simulink model "mavlinkMST"  (R2025b)
settings: Solver=ode1  StartTime=0.0  StopTime=inf  FixedStep=0.01  RelTol=1e-3
libraries: instrumentlib x2, uavmavlinklib x1
settings Model: Creator=y3353li  LastModifiedBy=yangli
settings DebuggingCC: UnderspecifiedInitializationDetection=Classic  MergeDetectMultiDrivingBlocksExec=none
settings ModelReferenceCC: PropagateSignalLabelsOutOfModel=off

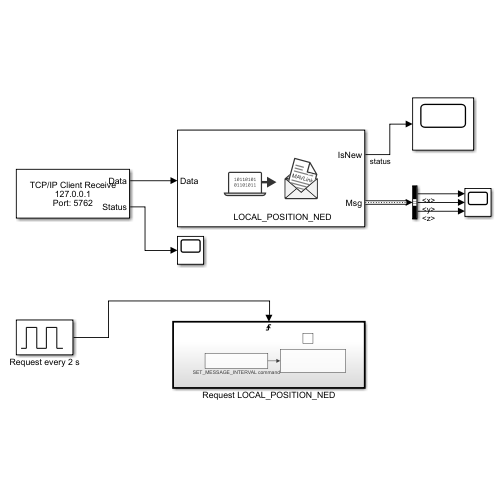
[thumbnail: Simulink's stored preview of the top-level diagram]
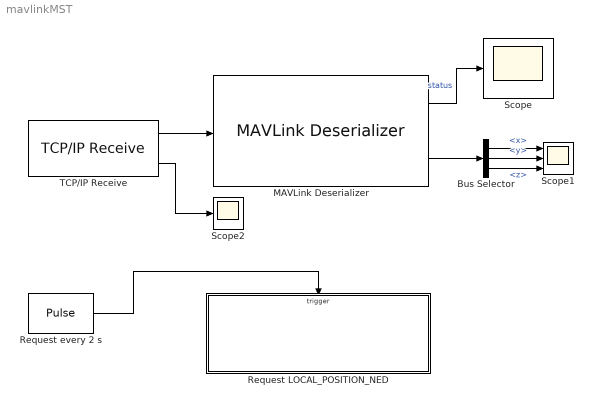
== system mavlinkMST ==
  Bus Selector : BusSelector  OutputSignals=Payload.x,Payload.y,Payload.z
  MAVLink Deserializer : uavmavlinklib/MAVLink Deserializer  dialectSource=Select from standard MAVLink dialects  dialect=common.xml  dialectCustom=common.xml  version=2  messageType=LOCAL_POSITION_NED  inputDataLength=off  SystemIDFilter=off  systemID=1  ComponentIDFilter=off  componentID=1  queueMsg=off  queueMsgSize=50  dropNum=off
  Request LOCAL_POSITION_NED : Subsystem  TreatAsAtomicUnit=on
  Request every 2 s : DiscretePulseGenerator  PulseType=Time based  PhaseDelay=0.1  SampleTime=0.01
  Scope : Scope
      settings: ActiveDisplayYMinimum=-1  ActiveDisplayYMaximum=1
  Scope1 : Scope  NumInputPorts=3
      settings: ActiveDisplayYMinimum=-75.175605297088623  ActiveDisplayYMaximum=89.282588481903076
  Scope2 : Scope
      settings: ActiveDisplayYMinimum=-1  ActiveDisplayYMaximum=1  DataLoggingVariableName=ScopeData2
  TCP/IP Receive : instrumentlib/TCP//IP Receive  Host=127.0.0.1  Port=5762  DataSize=64  DataType=uint8  ASCIIFormatting=%f  Terminator=LF  CustomTerminator=10  ByteOrder=big-endian  EnableBlockingMode=off  Timeout=10  SampleTime=0.01  SimulateUsing=Interpreted execution
  wires:
  MAVLink Deserializer/1 -> Scope/1  "status"
  MAVLink Deserializer/2 -> Bus Selector/1
  TCP/IP Receive/1 -> MAVLink Deserializer/1
  TCP/IP Receive/2 -> Scope2/1
  Request every 2 s/1 -> Request LOCAL_POSITION_NED/Trigger
  Bus Selector/1 -> Scope1/1  "<x>"
  Bus Selector/2 -> Scope1/2  "<y>"
  Bus Selector/3 -> Scope1/3  "<z>"

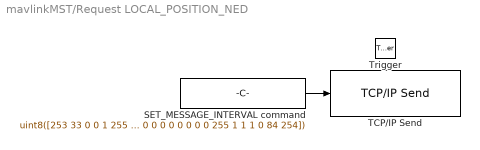
== system mavlinkMST/Request LOCAL_POSITION_NED ==
  Trigger : TriggerPort  VariantControl=(inherit)
  SET_MESSAGE_INTERVAL command : Constant  Value=uint8([253 33 0 0 1 255 190 76 0 0 0 0 0 66 0 80 195 71 0 0 0 0 0 0 0 0 0 0 0 0 0 0 0 0 0 0 0 0 255 1 1 1 0 84 254])
  TCP/IP Send : instrumentlib/TCP//IP Send  Host=127.0.0.1  Port=5762  ByteOrder=big-endian  EnableBlockingMode=on  Timeout=2  TransferDelay=off  SimulateUsing=Interpreted execution
  wires:
  SET_MESSAGE_INTERVAL command/1 -> TCP/IP Send/1
